simulink model "discrete_2d_lab1FDD"  (Simulink 9.0)
settings: Solver=ode5  StartTime=0.0  StopTime=15  FixedStep=0.025  RelTol=1e-3  EnableMultiTasking=on
values from neighbouring files (symbols this model uses):
  A1 = [0.976894729302  0.00384928405315; 0.0935733769434  0.922488606822]    [A1B1.mat]
  B1 = [2.15211975239 3.81864228746]    [A1B1.mat]
libraries: simulink x3
settings Model: Creator=b1048743  LastModifiedBy=Tom
settings DataIOCC: LimitDataPoints=on  SignalLoggingSaveFormat=ModelDataLogs  SignalLoggingName=sigsOut
settings OptimizationCC: BlockReduction=off  BooleanDataType=off  LifeSpan=auto
settings DebuggingCC: SaveWithParameterizedLinksMsg=none  SignalResolutionControl=TryResolveAllWithWarning  MultiTaskDSMMsg=warning  MultiTaskCondExecSysMsg=none  SFUnexpectedBacktrackingDiag=error  SFNoUnconditionalDefaultTransitionDiag=error  SFExecutionAtInitializationDiag=warning
settings HardwareCC: TargetUnknown=on
settings GRTTargetCC: CombineOutputUpdateFcns=off  GRTInterface=on

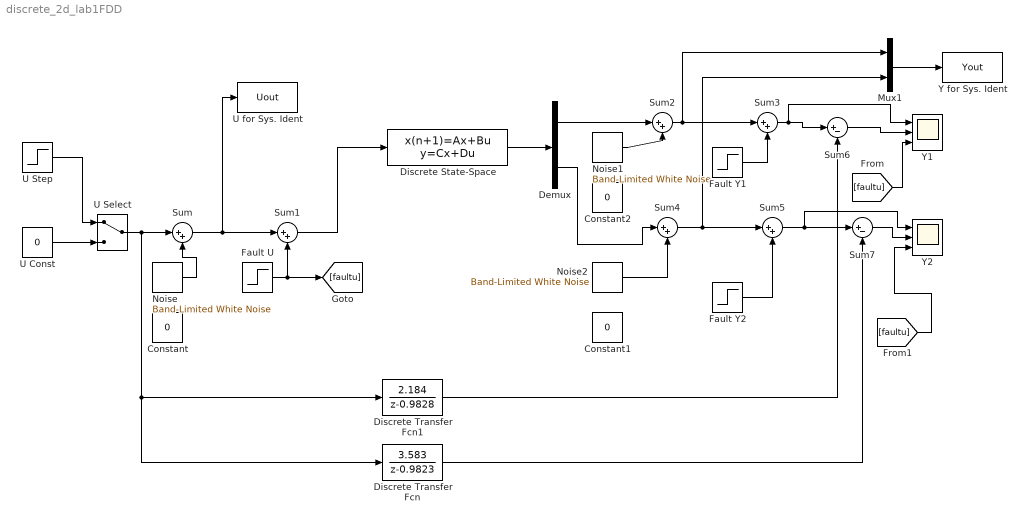
== system discrete_2d_lab1FDD ==
  Constant : Constant  Value=0
  Constant1 : Constant  Value=0
  Constant2 : Constant  Value=0
  Demux : Demux  Outputs=2
  Discrete Transfer Fcn : DiscreteTransferFcn  Numerator=[3.583]  Denominator=[1 -0.9823]
  Discrete Transfer Fcn1 : DiscreteTransferFcn  Numerator=[2.184]  Denominator=[1 -0.9828]
  Discrete State-Space : DiscreteStateSpace  A=A1  B=B1  C=[1 0; 0 1]  D=[0;0]  SampleTime=0.025
  Fault U : Step  Time=5  After=0  SampleTime=0
  Fault Y1 : Step  Time=3  After=0  SampleTime=0
  Fault Y2 : Step  After=0  SampleTime=0
  Mux1 : Mux  Inputs=2
  Noise : simulink/Sources/Band-Limited White Noise  Cov=[0.01]  Ts=0.025  seed=[23341]
  Noise1 : simulink/Sources/Band-Limited White Noise  Cov=[0.1]  Ts=0.025  seed=[23341]
  Noise2 : simulink/Sources/Band-Limited White Noise  Cov=[0.1]  Ts=0.025  seed=[23341]
  Sum{,1..5} (6 alike) : Sum  Inputs=|++  SaturateOnIntegerOverflow=on
  Sum6 : Sum  Inputs=|+-
  Sum7 : Sum  Inputs=|+-
  U Const : Constant  Value=0
  "U Select " : ManualSwitch
  U Step : Step  SampleTime=0
  U for Sys. Ident : ToWorkspace  VariableName=Uout  SampleTime=0.025
  Y for Sys. Ident : ToWorkspace  VariableName=Yout  SampleTime=0.025
  Y1 : Scope  NumInputPorts=3
  Y2 : Scope  NumInputPorts=3
  wires:
  U Const/1 -> "U Select "/2
  U Step/1 -> "U Select "/1
  Mux1/1 -> Y for Sys. Ident/1
  Discrete State-Space/1 -> Demux/1
  Sum1/1 -> Discrete State-Space/1
  Fault U/1 -> [faultu], Sum1/2
  Sum2/1 -> Sum3/1, Mux1/1
  Fault Y1/1 -> Sum3/2
  Sum4/1 -> Sum5/1, Mux1/2
  Fault Y2/1 -> Sum5/2
  Demux/1 -> Sum2/1
  Demux/2 -> Sum4/1
  Sum/1 -> Sum1/1, U for Sys. Ident/1
  "U Select "/1 -> Discrete Transfer Fcn1/1, Discrete Transfer Fcn/1, Sum/1
  Sum3/1 -> Y1/1, Sum6/1
  Discrete Transfer Fcn1/1 -> Sum6/2
  Sum5/1 -> Y2/1, Sum7/1
  Discrete Transfer Fcn/1 -> Sum7/2
  [faultu] -> Y1/3
  [faultu] -> Y2/3
  Noise/1 -> Sum/2
  Noise1/1 -> Sum2/2
  Noise2/1 -> Sum4/2
  Sum6/1 -> Y1/2
  Sum7/1 -> Y2/2
